simulink model "Admittance_Control"  (R2020b)
settings: Solver=VariableStepAuto  StartTime=0.0  StopTime=tk(end)-tk(1)  RelTol=1e-3
values from neighbouring files (symbols this model uses):
  B = myRobot.B_Lagrangian    [hw13_main.m]
  C = myRobot.C_Lagrangian    [hw13_main.m]
  dJa = myRobot.dJa    [hw13_main.m]
  F = myRobot.F    [hw13_main.m]
  G = myRobot.G_Lagrangian    [hw13_main.m]
  Ja = myRobot.Ja    [hw13_main.m]
  Ja_inv = pinv(Ja)    [hw13_main.m]
  K = diag([1,10,1,0,0,0])    [hw13_main.m]
  Kd = diag([240,15,150,0,0,0])    [hw13_main.m]
  KDt = diag([1 3 1 1 1 1]).*10    [hw13_main.m]
  Kp = diag([28,22,20,0,0,0])    [hw13_main.m]
  KPt = diag([1 0.1 1 1 1 1]).*100    [hw13_main.m]
  Mt = diag([1 1 1 1 1 1])    [hw13_main.m]
  Ts = 0.001    [hw13_main.m]
  x_r = [0.3;0.26; 0.3; -pi/2; -pi/2; -pi/2]    [hw13_main.m]
settings Model: Creator=nicol  LastModifiedBy=nicol

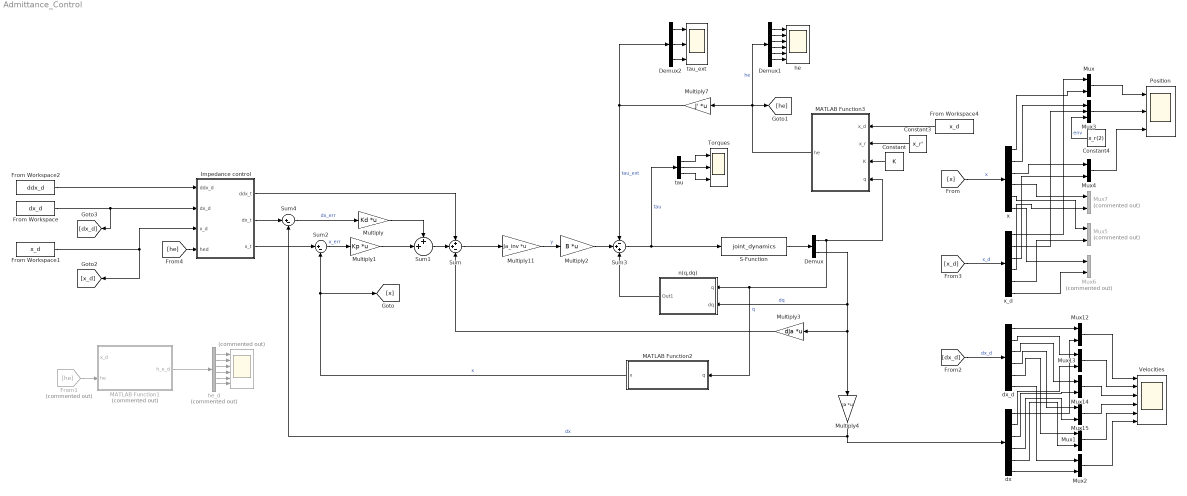
== system Admittance_Control ==
  " " : Scope  Commented=on  NumInputPorts=6
  Constant : Constant  Value=K
  Constant3 : Constant  Value=x_r'
  Constant4 : Constant  Value=x_r(2)
  Demux : Demux  Outputs=2
  Demux1 : Demux  Outputs=6
  Demux2 : Demux  Outputs=3
  From Workspace : FromWorkspace  VariableName=dx_d  SampleTime=Ts
  From Workspace1 : FromWorkspace  VariableName=x_d  SampleTime=Ts
  From Workspace2 : FromWorkspace  VariableName=ddx_d  SampleTime=Ts
  From Workspace4 : FromWorkspace  VariableName=x_d  SampleTime=Ts
  From1 : From  Commented=on  GotoTag=he
  Impedance control : Subsystem
  MATLAB Function1 : MATLAB Function  Commented=on  TreatAsAtomicUnit=on
  MATLAB Function2 : MATLAB Function  TreatAsAtomicUnit=on
  MATLAB Function3 : MATLAB Function  TreatAsAtomicUnit=on
  Multiply : Gain  Gain=Kd  Multiplication=Matrix(K*u)
  Multiply1 : Gain  Gain=Kp  Multiplication=Matrix(K*u)
  Multiply11 : Gain  Gain=Ja_inv  Multiplication=Matrix(K*u)
  Multiply2 : Gain  Gain=B  Multiplication=Matrix(K*u)
  Multiply3 : Gain  Gain=dJa  Multiplication=Matrix(K*u)
  Multiply4 : Gain  Gain=Ja  Multiplication=Matrix(K*u)
  Multiply7 : Gain  Gain=J'  Multiplication=Matrix(K*u)
  Mux{,1..2,4,12..15} (8 alike) : Mux  Inputs=2
  Mux3 : Mux  Inputs=3
  Mux5 : Mux  Commented=on  Inputs=2
  Mux6 : Mux  Commented=on  Inputs=2
  Mux7 : Mux  Commented=on  Inputs=2
  Position : Scope  NumInputPorts=3
  S-Function : S-Function  FunctionName=joint_dynamics  Parameters=myRobot  SFunctionDeploymentMode=off  EnableBusSupport=off
  Sum : Sum  Inputs=++-
  Sum1 : Sum  Inputs=++|
  Sum2 : Sum  Inputs=|+-
  Sum3 : Sum  Inputs=-++
  Sum4 : Sum  Inputs=|+-
  Torques : Scope  NumInputPorts=3
  Velocities : Scope  NumInputPorts=6
  dx : Demux  Outputs=6
  dx_d : Demux  Outputs=6
  he : Scope  NumInputPorts=6
  he_d : Demux  Commented=on  Outputs=6
  n(q,dq) : Subsystem
  tau : Demux  Outputs=3
  tau_ext : Scope  NumInputPorts=3
  x : Demux  Outputs=6
  x_d : Demux  Outputs=6
  wires:
  MATLAB Function1/1(h_e_d) -> he_d/1
  From Workspace/1 -> [dx_d], Impedance control/2(dx_d)
  From Workspace2/1 -> Impedance control/1(ddx_d)
  MATLAB Function2/1(x) -> Sum2/2, [x]  "x"
  Demux/2 -> n(q,dq)/2(dq), Multiply3/1, Multiply4/1  "dq"
  n(q,dq)/1(Out1) -> Sum3/3
  Sum3/1 -> tau/1, S-Function/1  "tau"
  Multiply4/1 -> Sum4/2, dx/1  "dx"
  Sum2/1 -> Multiply1/1  "x_err"
  Multiply2/1 -> Sum3/2
  S-Function/1 -> Demux/1
  Multiply1/1 -> Sum1/2
  Multiply/1 -> Sum1/1
  Demux/1 -> MATLAB Function3/4(q), n(q,dq)/1(q), MATLAB Function2/1(q)  "q"
  Demux2/3 -> tau_ext/3
  Multiply7/1 -> Sum3/1, Demux2/1  "tau_ext"
  Demux2/2 -> tau_ext/2
  Demux1/4 -> he/4
  Demux1/5 -> he/5
  Demux1/6 -> he/6
  Demux1/3 -> he/3
  Demux2/1 -> tau_ext/1
  Demux1/2 -> he/2
  Demux1/1 -> he/1
  From1/1 -> MATLAB Function1/2(he)
  tau/2 -> Torques/2
  tau/1 -> Torques/1
  tau/3 -> Torques/3
  From Workspace1/1 -> [x_d], Impedance control/3(x_d)
  [x_d] -> x_d/1  "x_d"
  [x] -> x/1  "x"
  dx_d/3 -> Mux14/1
  dx/2 -> Mux13/2
  dx_d/4 -> Mux15/1
  dx/6 -> Mux2/2
  dx/1 -> Mux12/2
  Mux1/1 -> Velocities/5
  dx_d/1 -> Mux12/1
  dx/3 -> Mux14/2
  Mux14/1 -> Velocities/3
  Mux12/1 -> Velocities/1
  dx_d/5 -> Mux1/1
  dx/4 -> Mux15/2
  dx/5 -> Mux1/2
  Mux2/1 -> Velocities/6
  dx_d/6 -> Mux2/1
  Mux15/1 -> Velocities/4
  dx_d/2 -> Mux13/1
  Mux13/1 -> Velocities/2
  [dx_d] -> dx_d/1  "dx_d"
  Multiply3/1 -> Sum/3
  Sum4/1 -> Multiply/1  "dx_err"
  Sum1/1 -> Sum/2
  Impedance control/2(dx_t) -> Sum4/1
  Impedance control/1(ddx_t) -> Sum/1
  Multiply11/1 -> Multiply2/1  "y"
  Sum/1 -> Multiply11/1
  he_d/3 -> " "/3
  he_d/2 -> " "/2
  he_d/6 -> " "/6
  he_d/5 -> " "/5
  he_d/4 -> " "/4
  he_d/1 -> " "/1
  Impedance control/3(x_t) -> Sum2/1
  x/1 -> Mux/2
  x_d/1 -> Mux/1
  x/2 -> Mux3/1
  x_d/2 -> Mux3/2
  x/3 -> Mux4/1
  x_d/3 -> Mux4/2
  x/4 -> Mux7/1
  x_d/4 -> Mux7/2
  x/5 -> Mux5/1
  x_d/5 -> Mux5/2
  x/6 -> Mux6/1
  x_d/6 -> Mux6/2
  Mux/1 -> Position/1
  Mux3/1 -> Position/2
  Mux4/1 -> Position/3
  Constant4/1 -> Mux3/3  "env"
  Constant3/1 -> MATLAB Function3/2(x_r)
  From Workspace4/1 -> MATLAB Function3/1(x_d)
  Constant/1 -> MATLAB Function3/3(K)
  [he] -> Impedance control/4(hed)
  MATLAB Function3/1(he) -> [he], Demux1/1, Multiply7/1  "he"

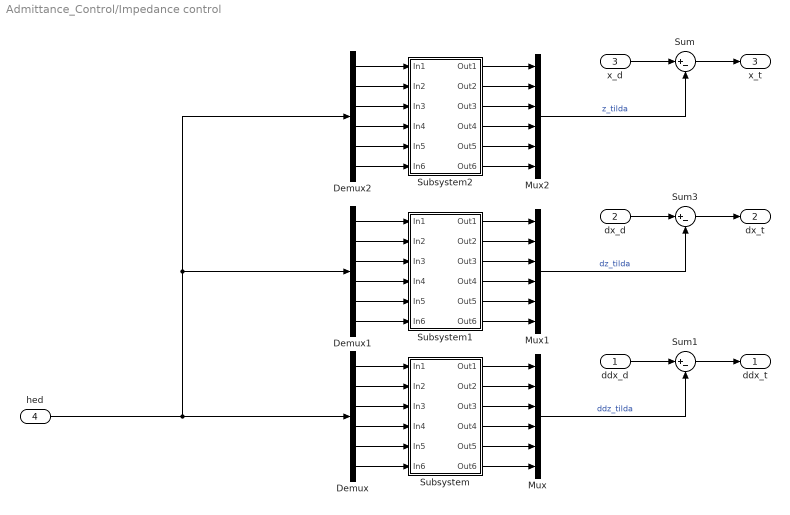
== system Admittance_Control/Impedance control ==
  ddx_d : Inport
  dx_d : Inport  Port=2
  x_d : Inport  Port=3
  hed : Inport  Port=4
  Demux : Demux  Outputs=6
  Demux1 : Demux  Outputs=6
  Demux2 : Demux  Outputs=6
  Mux : Mux  Inputs=6
  Mux1 : Mux  Inputs=6
  Mux2 : Mux  Inputs=6
  Subsystem : Subsystem
  Subsystem1 : Subsystem
  Subsystem2 : Subsystem
  Sum : Sum  Inputs=|+-
  Sum1 : Sum  Inputs=|+-
  Sum3 : Sum  Inputs=|+-
  ddx_t : Outport
  dx_t : Outport  Port=2
  x_t : Outport  Port=3
  wires:
  hed/1 -> Demux2/1, Demux1/1, Demux/1
  Sum1/1 -> ddx_t/1
  Sum/1 -> x_t/1
  Sum3/1 -> dx_t/1
  dx_d/1 -> Sum3/1
  ddx_d/1 -> Sum1/1
  x_d/1 -> Sum/1
  Mux/1 -> Sum1/2  "ddz_tilda"
  Demux/1 -> Subsystem/1(In1)
  Demux/2 -> Subsystem/2(In2)
  Demux/3 -> Subsystem/3(In3)
  Demux/4 -> Subsystem/4(In4)
  Demux/5 -> Subsystem/5(In5)
  Demux/6 -> Subsystem/6(In6)
  Subsystem/1(Out1) -> Mux/1
  Subsystem/2(Out2) -> Mux/2
  Subsystem/3(Out3) -> Mux/3
  Subsystem/4(Out4) -> Mux/4
  Subsystem/5(Out5) -> Mux/5
  Subsystem/6(Out6) -> Mux/6
  Subsystem1/6(Out6) -> Mux1/6
  Subsystem1/5(Out5) -> Mux1/5
  Subsystem1/4(Out4) -> Mux1/4
  Subsystem1/1(Out1) -> Mux1/1
  Demux1/6 -> Subsystem1/6(In6)
  Subsystem1/3(Out3) -> Mux1/3
  Demux1/3 -> Subsystem1/3(In3)
  Demux1/5 -> Subsystem1/5(In5)
  Demux1/4 -> Subsystem1/4(In4)
  Demux1/2 -> Subsystem1/2(In2)
  Demux1/1 -> Subsystem1/1(In1)
  Subsystem1/2(Out2) -> Mux1/2
  Subsystem2/6(Out6) -> Mux2/6
  Subsystem2/5(Out5) -> Mux2/5
  Subsystem2/4(Out4) -> Mux2/4
  Subsystem2/1(Out1) -> Mux2/1
  Demux2/6 -> Subsystem2/6(In6)
  Subsystem2/3(Out3) -> Mux2/3
  Demux2/3 -> Subsystem2/3(In3)
  Demux2/5 -> Subsystem2/5(In5)
  Demux2/4 -> Subsystem2/4(In4)
  Demux2/2 -> Subsystem2/2(In2)
  Demux2/1 -> Subsystem2/1(In1)
  Subsystem2/2(Out2) -> Mux2/2
  Mux1/1 -> Sum3/2  "dz_tilda"
  Mux2/1 -> Sum/2  "z_tilda"

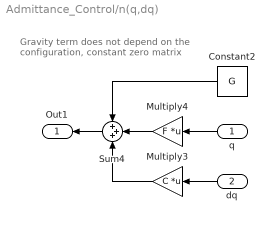
== system Admittance_Control/n(q,dq) ==
  note: Gravity term does not depend on the
      |  configuration, constant zero matrix
  q : Inport
  dq : Inport  Port=2
  Constant2 : Constant  Value=G  VectorParams1D=off
  Multiply3 : Gain  Gain=C  Multiplication=Matrix(K*u)
  Multiply4 : Gain  Gain=F  Multiplication=Matrix(K*u)
  Sum4 : Sum  Inputs=+++
  Out1 : Outport
  wires:
  Sum4/1 -> Out1/1
  Multiply3/1 -> Sum4/3
  Multiply4/1 -> Sum4/2
  Constant2/1 -> Sum4/1
  q/1 -> Multiply4/1
  dq/1 -> Multiply3/1

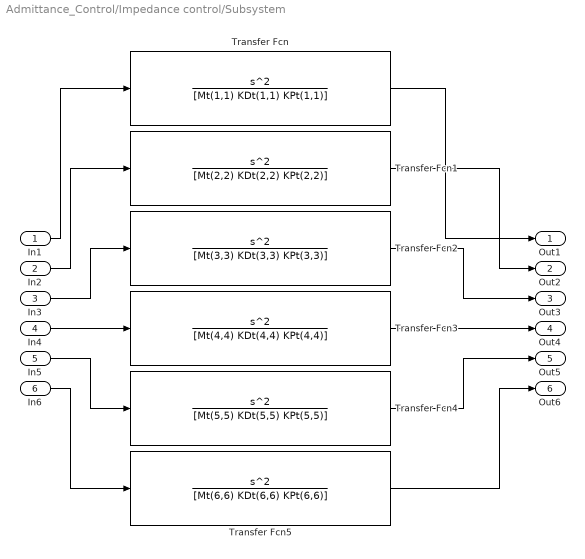
== system Admittance_Control/Impedance control/Subsystem ==
  In1 : Inport
  In2 : Inport  Port=2
  In3 : Inport  Port=3
  In4 : Inport  Port=4
  In5 : Inport  Port=5
  In6 : Inport  Port=6
  Transfer Fcn : TransferFcn  Numerator=[1 0 0]  Denominator=[Mt(1,1) KDt(1,1) KPt(1,1)]
  Transfer Fcn1 : TransferFcn  Numerator=[1 0 0]  Denominator=[Mt(2,2) KDt(2,2) KPt(2,2)]
  Transfer Fcn2 : TransferFcn  Numerator=[1 0 0]  Denominator=[Mt(3,3) KDt(3,3) KPt(3,3)]
  Transfer Fcn3 : TransferFcn  Numerator=[1 0 0]  Denominator=[Mt(4,4) KDt(4,4) KPt(4,4)]
  Transfer Fcn4 : TransferFcn  Numerator=[1 0 0]  Denominator=[Mt(5,5) KDt(5,5) KPt(5,5)]
  Transfer Fcn5 : TransferFcn  Numerator=[1 0 0]  Denominator=[Mt(6,6) KDt(6,6) KPt(6,6)]
  Out1 : Outport
  Out2 : Outport  Port=2
  Out3 : Outport  Port=3
  Out4 : Outport  Port=4
  Out5 : Outport  Port=5
  Out6 : Outport  Port=6
  wires:
  In4/1 -> Transfer Fcn3/1
  In2/1 -> Transfer Fcn1/1
  Transfer Fcn1/1 -> Out2/1
  In6/1 -> Transfer Fcn5/1
  Transfer Fcn4/1 -> Out5/1
  Transfer Fcn2/1 -> Out3/1
  In5/1 -> Transfer Fcn4/1
  In1/1 -> Transfer Fcn/1
  Transfer Fcn3/1 -> Out4/1
  In3/1 -> Transfer Fcn2/1
  Transfer Fcn5/1 -> Out6/1
  Transfer Fcn/1 -> Out1/1

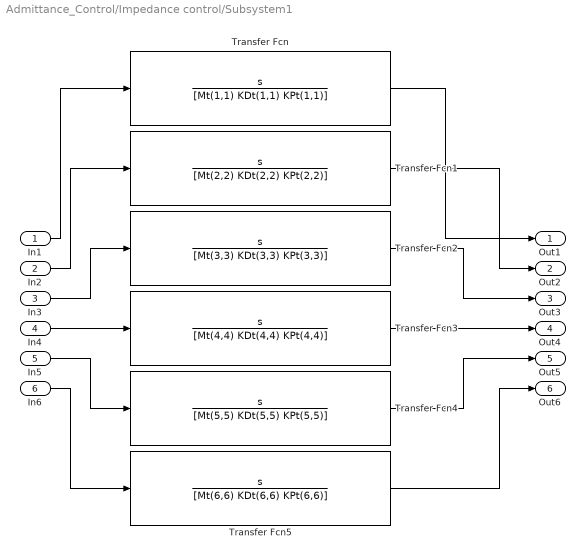
== system Admittance_Control/Impedance control/Subsystem1 ==
  In1 : Inport
  In2 : Inport  Port=2
  In3 : Inport  Port=3
  In4 : Inport  Port=4
  In5 : Inport  Port=5
  In6 : Inport  Port=6
  Transfer Fcn : TransferFcn  Numerator=[0 1 0]  Denominator=[Mt(1,1) KDt(1,1) KPt(1,1)]
  Transfer Fcn1 : TransferFcn  Numerator=[0 1 0]  Denominator=[Mt(2,2) KDt(2,2) KPt(2,2)]
  Transfer Fcn2 : TransferFcn  Numerator=[0 1 0]  Denominator=[Mt(3,3) KDt(3,3) KPt(3,3)]
  Transfer Fcn3 : TransferFcn  Numerator=[0 1 0]  Denominator=[Mt(4,4) KDt(4,4) KPt(4,4)]
  Transfer Fcn4 : TransferFcn  Numerator=[0 1 0]  Denominator=[Mt(5,5) KDt(5,5) KPt(5,5)]
  Transfer Fcn5 : TransferFcn  Numerator=[0 1 0]  Denominator=[Mt(6,6) KDt(6,6) KPt(6,6)]
  Out1 : Outport
  Out2 : Outport  Port=2
  Out3 : Outport  Port=3
  Out4 : Outport  Port=4
  Out5 : Outport  Port=5
  Out6 : Outport  Port=6
  wires:
  In4/1 -> Transfer Fcn3/1
  In2/1 -> Transfer Fcn1/1
  Transfer Fcn1/1 -> Out2/1
  In6/1 -> Transfer Fcn5/1
  Transfer Fcn4/1 -> Out5/1
  Transfer Fcn2/1 -> Out3/1
  In5/1 -> Transfer Fcn4/1
  In1/1 -> Transfer Fcn/1
  Transfer Fcn3/1 -> Out4/1
  In3/1 -> Transfer Fcn2/1
  Transfer Fcn5/1 -> Out6/1
  Transfer Fcn/1 -> Out1/1

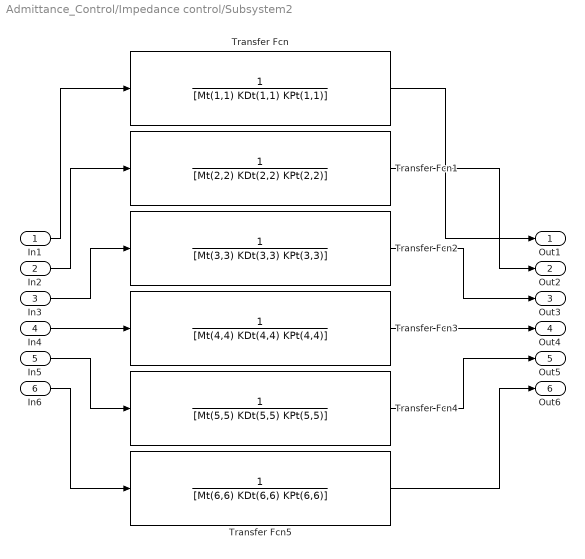
== system Admittance_Control/Impedance control/Subsystem2 ==
  In1 : Inport
  In2 : Inport  Port=2
  In3 : Inport  Port=3
  In4 : Inport  Port=4
  In5 : Inport  Port=5
  In6 : Inport  Port=6
  Transfer Fcn : TransferFcn  Numerator=[0 0 1]  Denominator=[Mt(1,1) KDt(1,1) KPt(1,1)]
  Transfer Fcn1 : TransferFcn  Numerator=[0 0 1]  Denominator=[Mt(2,2) KDt(2,2) KPt(2,2)]
  Transfer Fcn2 : TransferFcn  Numerator=[0 0 1]  Denominator=[Mt(3,3) KDt(3,3) KPt(3,3)]
  Transfer Fcn3 : TransferFcn  Numerator=[0 0 1]  Denominator=[Mt(4,4) KDt(4,4) KPt(4,4)]
  Transfer Fcn4 : TransferFcn  Numerator=[0 0 1]  Denominator=[Mt(5,5) KDt(5,5) KPt(5,5)]
  Transfer Fcn5 : TransferFcn  Numerator=[0 0 1]  Denominator=[Mt(6,6) KDt(6,6) KPt(6,6)]
  Out1 : Outport
  Out2 : Outport  Port=2
  Out3 : Outport  Port=3
  Out4 : Outport  Port=4
  Out5 : Outport  Port=5
  Out6 : Outport  Port=6
  wires:
  In4/1 -> Transfer Fcn3/1
  In2/1 -> Transfer Fcn1/1
  Transfer Fcn1/1 -> Out2/1
  In6/1 -> Transfer Fcn5/1
  Transfer Fcn4/1 -> Out5/1
  Transfer Fcn2/1 -> Out3/1
  In5/1 -> Transfer Fcn4/1
  In1/1 -> Transfer Fcn/1
  Transfer Fcn3/1 -> Out4/1
  In3/1 -> Transfer Fcn2/1
  Transfer Fcn5/1 -> Out6/1
  Transfer Fcn/1 -> Out1/1

== matlab function Admittance_Control/MATLAB Function1 ==
  data: x_d input; he input; h_e_d output
function h_e_d = getH_e_d(x_d, he)

phi_d=x_d(4:6,1);
R_d=eul2rotm(phi_d','ZYZ');

f_e_d=R_d'*he(1:3,1);
tau_e_d=R_d'*he(4:6,1);
h_e_d=[f_e_d;tau_e_d];

% Ta=getTa(phi_d(1),phi_d(2),phi_d(3));
% h_e_d=Ta'*he;

end

== matlab function Admittance_Control/MATLAB Function3 ==
  data: x_d input; x_r input; K input; q input; he output
function he = Environment(x_d,x_r,K,q)

T_e=getTe(q);
x_e=zeros(6,1);
x_e(1:3,1)=T_e(1:3,4);
eul_e = rotm2eul(T_e(1:3,1:3),'ZYZ');
x_e(4:6,1)=eul_e;

if(x_e(2,1)-x_r(2,1)<0)
    he=[0;0;0;0;0;0];
else
    sup=zeros(6,1);
    dx_r_d=x_d-x_r;
    dx_e_d=x_d-x_e;
    sup(2,1)=dx_r_d(2,1)-dx_e_d(2,1);
    he=K*sup;
end

== matlab function Admittance_Control/MATLAB Function2 ==
  data: q input size=3; x output size=6
function x = directKinematics6Dof(q)
%last 3 components assigned constant since robot does not have rotational
%joints

x=[ q(1) + 1/5;
    q(3) + 1/5;
    q(2) + 1251/5000;
    -pi/2;
    -pi/2;
    -pi/2];
end
